simulink model "GridConnectedPVarray"  (R2024a)
settings: Solver=VariableStepAuto  StartTime=0.0  StopTime=1  RelTol=1e-3
libraries: spsSeriesRLCBranchLib x13, spsDiodeLib x7, spsIGBTDiodeLib x7, spsMeanLib x3, spsThreePhaseVIMeasurementLib x3, spsVoltageMeasurementLib x2, slpidlib x2, spsCurrentMeasurementLib x1, spsPVArrayLib x1, simulink x1, eeGeneralControl x1, spsThreePhaseSourceLib x1
settings Model: Creator=aditl  LastModifiedBy=aditl

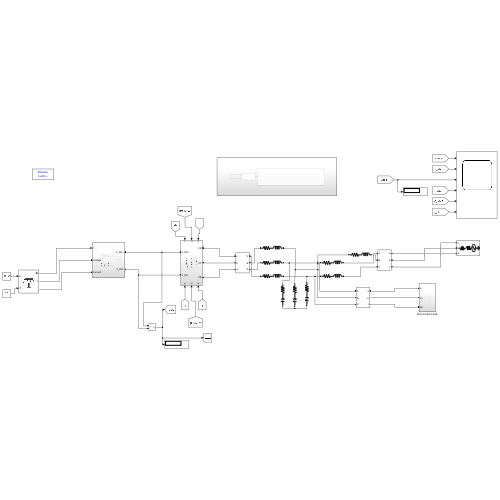
[thumbnail: Simulink's stored preview of the top-level diagram]
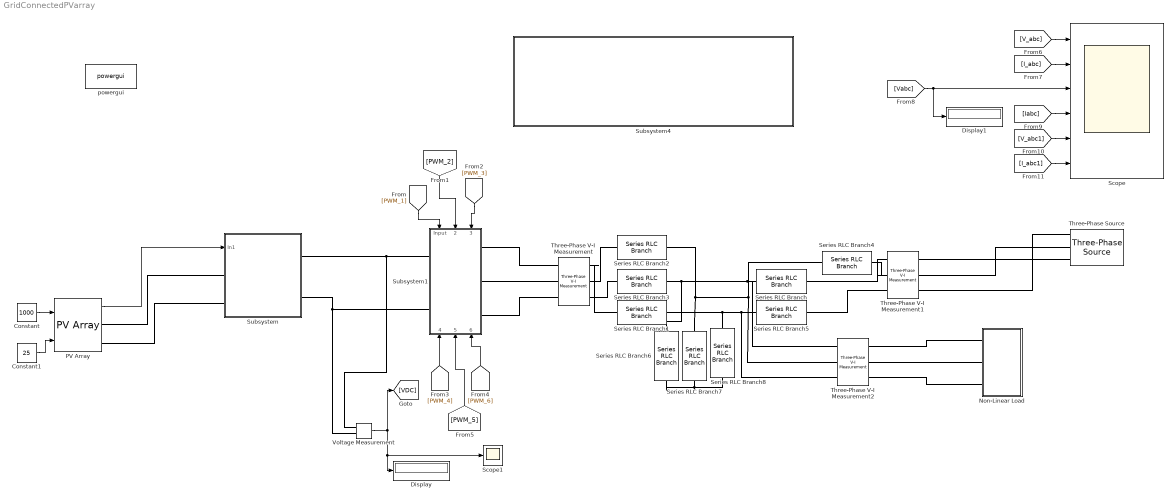
== system GridConnectedPVarray ==
  Constant : Constant  Value=1000
  Constant1 : Constant  Value=25
  Display : Display
  Display1 : Display
  Non-Linear Load : Subsystem
  PV Array : spsPVArrayLib/PV Array  Npar=40  Nser=10  PlotType=array @ 1000 W/m2 & specified temperatures  S_vec="[ 1000  500  100 ]"  Temp_C_vec="[ 45 25  ]"  ModuleName=User-defined  PlotWhenSelected=off  Pm=213.15  Ncell=60  Voc=36.3  Isc=7.84  Vm=29  Im=7.35  beta_Voc_pc=-0.36099  alpha_Isc_pc=0.102  beta_Voc=-0.13104  alpha_Isc=0.0079968  IL=7.8654  I0=2.9273e-10  nI=0.98119  Rsh=313.0553  Rs=0.39381  RobustModel=off  RobustCellTemperature=313.3991  BAL=on  Tc=1e-6  Tfilter=5e-5
  Scope : Scope  NumInputPorts=6
  Scope1 : Scope
  Series RLC Branch{,1..5} (6 alike) : spsSeriesRLCBranchLib/Series RLC Branch  LConnTagsString=__new0  RConnTagsString=__new0  BranchType=RL  Resistance=1e-3  Inductance=500e-6  SetiL0=off  InitialCurrent=0  Capacitance=1e-6  Setx0=off  InitialVoltage=0  Measurements=None
  Series RLC Branch6 : spsSeriesRLCBranchLib/Series RLC Branch  LConnTagsString=__new0  RConnTagsString=__new0  BranchType=RC  Resistance=1e-3  Inductance=1e-3  SetiL0=off  InitialCurrent=0  Capacitance=100e-6  Setx0=off  InitialVoltage=0  Measurements=None
  Series RLC Branch7 : spsSeriesRLCBranchLib/Series RLC Branch  LConnTagsString=__new0  RConnTagsString=__new0  BranchType=RC  Resistance=1e-3  Inductance=1e-3  SetiL0=off  InitialCurrent=0  Capacitance=100e-6  Setx0=off  InitialVoltage=0  Measurements=None
  Series RLC Branch8 : spsSeriesRLCBranchLib/Series RLC Branch  LConnTagsString=__new0  RConnTagsString=__new0  BranchType=RC  Resistance=1e-3  Inductance=1e-3  SetiL0=off  InitialCurrent=0  Capacitance=100e-6  Setx0=off  InitialVoltage=0  Measurements=None
  Subsystem : Subsystem
  Subsystem1 : Subsystem
      settings: PortSchema="{\"entries\":[{\"content\":{\"sides\":[{\"content\":{\"connectorIds\":[\"LConn1\",\"LConn2\"]},\"type\":\"ConnectorPlacement.EquallySpacedRectSide\",\"uuid\":\"a2a7ddac-ae87-4c1a-8b74-688f39786139\"},{\"content\":{\"connectorIds\":[\"RConn1\",\"RConn2\",\"RConn3\"],\"side\":\"RIGHT\"},\"type\":\"ConnectorPlacement.EquallySpacedRectSide\",\"uuid\":\"0ffaccab-b326-455c-8204-264bcaba31f0\"},{\"content\":{\"connectorIds\":[\"In1\",\"In2\",\"In3\"],\"side\":\"TOP\"},\"type\":\"ConnectorPlacement.EquallySpacedRectSide\",\"uuid\":\"7b315db4-04ed-4dc6-88af-8ad8e918cdd7\"},{\"content\":{\"connectorIds\":[\"In4\",\"In5\",\"In6\"],\"side\":\"BOTTOM\"},\"type\":\"ConnectorPlacement.EquallySpacedRectSide\",\"uuid\":\"b8aad6e0-d398-4abc-9931-0eadad765190\"}]},\"type\":\"ConnectorPlacement.EquallySpacedConnector\",\"uuid\":\"72918063-f98b-4253-8381-9410a0d32035\"}],\"packageUris\":[\"http://schema.mathworks.com/mf0/Connector/R2020b\"],\"version\":\"1.0\"}"
  Subsystem4 : Subsystem
  Three-Phase V-I Measurement : spsThreePhaseVIMeasurementLib/Three-Phase V-I Measurement  VoltageMeasurement=phase-to-ground  SetLabelV=on  LabelV=V_abc  Vpu=off  VpuLL=off  CurrentMeasurement=yes  SetLabelI=on  LabelI=I_abc  Ipu=off  Pbase=100e6  Vbase=500e3  OutputType=Complex  PhasorSimulation=off  PSBequivalent=0
  Three-Phase V-I Measurement1 : spsThreePhaseVIMeasurementLib/Three-Phase V-I Measurement  VoltageMeasurement=phase-to-ground  SetLabelV=on  LabelV=Vabc  Vpu=off  VpuLL=off  CurrentMeasurement=yes  SetLabelI=on  LabelI=Iabc  Ipu=off  Pbase=100e6  Vbase=500e3  OutputType=Complex  PhasorSimulation=off  PSBequivalent=0
  Three-Phase V-I Measurement2 : spsThreePhaseVIMeasurementLib/Three-Phase V-I Measurement  VoltageMeasurement=phase-to-ground  SetLabelV=on  LabelV=V_abc1  Vpu=off  VpuLL=off  CurrentMeasurement=yes  SetLabelI=on  LabelI=I_abc1  Ipu=off  Pbase=100e6  Vbase=500e3  OutputType=Complex  PhasorSimulation=off  PSBequivalent=0
  Three-Phase Source : spsThreePhaseSourceLib/Three-Phase Source  InternalConnection=Yg  VoltagePhases=off  Voltage=415  PhaseAngle=0  Voltage_phases=[25e3 25e3 25e3]/sqrt(3)  PhaseAngles_phases=[0 -120 +120]  Frequency=50  NonIdealSource=on  SpecifyImpedance=off  Resistance=1e-6  Inductance=1e6  ShortCircuitLevel=100e6  BaseVoltage=400  XRratio=7  BusType=swing  Pref=10e3  Qref=0  Prefabc=[10e3, 10e3, 10e3]  Qrefabc=[0, 0, 0]  Qmin=-inf  Qmax=inf
  Voltage Measurement : spsVoltageMeasurementLib/Voltage Measurement  PhasorSimulation=off  OutputType=Complex  PSBequivalent=0
  powergui : spspowerguiLib/powergui  Priority=1  SimulationMode=Discrete  SampleTime=1e-06  frequency=60  Iterations=50  frequencyindice=0  Pbase=100e6  ErrMax=1e-4  UnitsV=kV  UnitsW=MW  buscounter=0  FunctionMessages=off  echomessages=off  EnableUseOfTLC=off  CurrentSourceSwitches=off  DisableSnubberDevices=off  DisableRonSwitches=off  DisableVfSwitches=off  DisplayEquations=off  AutomaticDiscreteSolvers=off  SolverType=Tustin/Backward Euler (TBE)  Interpol=off  ExternalGateDelay=off  methode=off  Ts=100  x0status=blocks  SPID=on  SwTol=0  HookPort=off  NonlinearTolerance=0  nMaxIteration=15  ContinueOnMaxIteration=off  RestoreLinks=warning  ResistiveCurrentMeasurement=off  Frange=[0:2:500]  Ylog=off  Xlog=on  ShowGrid=off  save=off  variable=ZData  structure=0  ZoomFFT=off  StartTime=0.0  cycles=1  DisplayStyle=1  fundamental=60  FreqAxis=off  MaxFrequency=1000  frequencyindicesteady=1  RmsSteady=1  display=off
  wires:
  Constant/1 -> PV Array/1
  Constant1/1 -> PV Array/2
  PV Array/1 -> Subsystem/1(In1)
  [PWM_1] -> Subsystem1/1(Input)
  [PWM_2] -> Subsystem1/2(Input1)
  [PWM_3] -> Subsystem1/3(Input2)
  [PWM_4] -> Subsystem1/4(Input3)
  [PWM_6] -> Subsystem1/6(Input4)
  [PWM_5] -> Subsystem1/5(Input5)
  [V_abc] -> Scope/1
  [I_abc] -> Scope/2
  [Vabc] -> Display1/1, Scope/3
  [Iabc] -> Scope/4
  [V_abc1] -> Scope/5
  [I_abc1] -> Scope/6
  Voltage Measurement/1 -> Scope1/1, Display/1, [VDC]
  connections:
  PV Array/RConn1 -- Subsystem/LConn1
  PV Array/RConn2 -- Subsystem/LConn2
  Subsystem1/LConn1 -- Voltage Measurement/LConn1 -- Subsystem/RConn1
  Subsystem1/LConn2 -- Voltage Measurement/LConn2 -- Subsystem/RConn2
  Series RLC Branch5/LConn1 -- Three-Phase V-I Measurement2/LConn3 -- Series RLC Branch8/LConn1 -- Series RLC Branch1/RConn1
  Series RLC Branch4/LConn1 -- Series RLC Branch7/LConn1 -- Series RLC Branch2/RConn1 -- Three-Phase V-I Measurement2/LConn2
  Series RLC Branch/LConn1 -- Three-Phase V-I Measurement2/LConn1 -- Series RLC Branch6/LConn1 -- Series RLC Branch3/RConn1
  Three-Phase V-I Measurement/RConn1 -- Subsystem1/RConn3
  Three-Phase V-I Measurement/RConn2 -- Subsystem1/RConn2
  Three-Phase V-I Measurement/RConn3 -- Subsystem1/RConn1
  Three-Phase V-I Measurement1/LConn1 -- Series RLC Branch/RConn1
  Three-Phase V-I Measurement1/LConn2 -- Series RLC Branch4/RConn1
  Three-Phase V-I Measurement1/LConn3 -- Series RLC Branch5/RConn1
  Series RLC Branch6/RConn1 -- Series RLC Branch7/RConn1 -- Series RLC Branch8/RConn1
  Three-Phase V-I Measurement2/RConn1 -- Non-Linear Load/LConn1
  Three-Phase V-I Measurement2/RConn2 -- Non-Linear Load/LConn2
  Three-Phase V-I Measurement2/RConn3 -- Non-Linear Load/LConn3
  Three-Phase V-I Measurement1/RConn1 -- Three-Phase Source/RConn1
  Three-Phase V-I Measurement1/RConn2 -- Three-Phase Source/RConn2
  Three-Phase Source/RConn3 -- Three-Phase V-I Measurement1/RConn3
  Three-Phase V-I Measurement/LConn1 -- Series RLC Branch3/LConn1
  Three-Phase V-I Measurement/LConn2 -- Series RLC Branch2/LConn1
  Three-Phase V-I Measurement/LConn3 -- Series RLC Branch1/LConn1

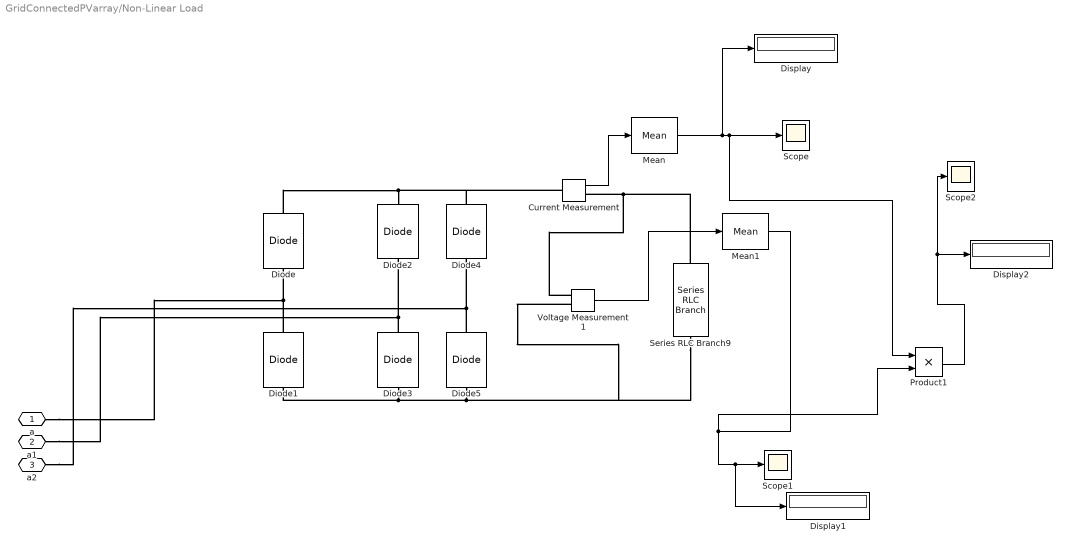
== system GridConnectedPVarray/Non-Linear Load ==
  Current Measurement : spsCurrentMeasurementLib/Current Measurement  PhasorSimulation=off  OutputType=Complex  PSBequivalent=0
  Diode{,1..5} (6 alike) : spsDiodeLib/Diode  Ron=0.001  Lon=0  Vf=0.8  IC=0  UseSnubber=0  Rs=500  Cs=250e-9  Measurements=off
  Display : Display
  Display1 : Display
  Display2 : Display
  Mean : spsMeanLib/Mean  Freq=60  Vinit=0  Ts=0
  Mean1 : spsMeanLib/Mean  Freq=60  Vinit=0  Ts=0
  Product1 : Product
  Scope : Scope
  Scope1 : Scope
  Scope2 : Scope
  Series RLC Branch9 : spsSeriesRLCBranchLib/Series RLC Branch  LConnTagsString=__new0  RConnTagsString=__new0  BranchType=RL  Resistance=31.23  Inductance=10e-3  SetiL0=off  InitialCurrent=0  Capacitance=1e-6  Setx0=off  InitialVoltage=0  Measurements=None
  Voltage Measurement1 : spsVoltageMeasurementLib/Voltage Measurement  PhasorSimulation=off  OutputType=Complex  PSBequivalent=0
  a : PMIOPort  Side=Left
  a1 : PMIOPort  Port=2  Side=Left
  a2 : PMIOPort  Port=3  Side=Left
  wires:
  Product1/1 -> Scope2/1, Display2/1
  Mean/1 -> Product1/1, Scope/1, Display/1
  Mean1/1 -> Display1/1, Scope1/1, Product1/2
  Voltage Measurement1/1 -> Mean1/1
  Current Measurement/1 -> Mean/1
  connections:
  Diode/RConn1 -- Current Measurement/LConn1 -- Diode4/RConn1 -- Diode2/RConn1
  Diode1/RConn1 -- Diode/LConn1 -- a/RConn1
  Diode3/LConn1 -- Voltage Measurement1/LConn2 -- Series RLC Branch9/RConn1 -- Diode5/LConn1 -- Diode1/LConn1
  Diode3/RConn1 -- Diode2/LConn1 -- a1/RConn1
  Diode5/RConn1 -- a2/RConn1 -- Diode4/LConn1
  Series RLC Branch9/LConn1 -- Voltage Measurement1/LConn1 -- Current Measurement/RConn1

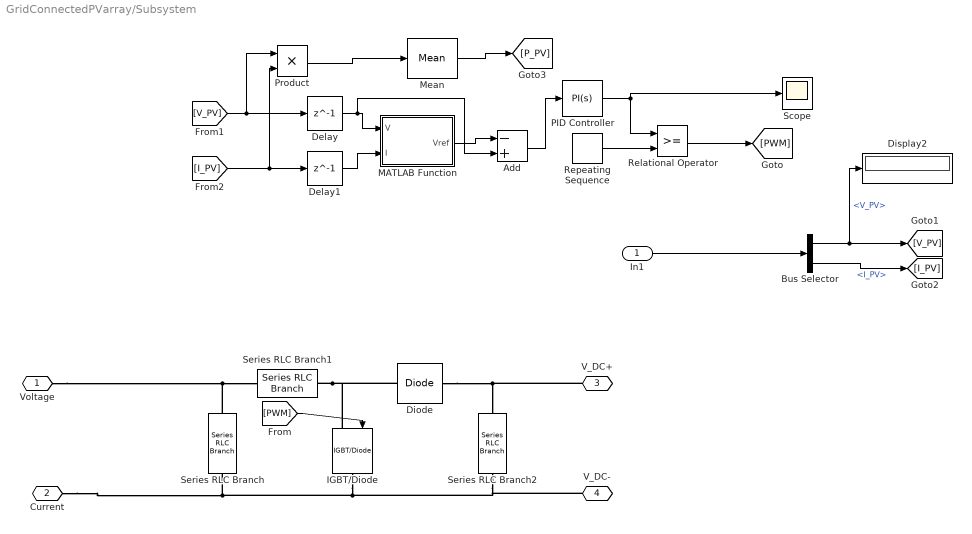
== system GridConnectedPVarray/Subsystem ==
  In1 : Inport
  Add : Sum  Inputs=-+
  Bus Selector : BusSelector  OutputSignals=V_PV,I_PV
  Delay : Delay  DelayLength=1  InitialCondition=0
  Delay1 : Delay  DelayLength=1  InitialCondition=0
  Diode : spsDiodeLib/Diode  Ron=0.001  Lon=2.2e-3  Vf=0.7  IC=0  UseSnubber=0  Rs=10e3  Cs=inf  Measurements=off
  Display2 : Display
  IGBT/Diode : spsIGBTDiodeLib/IGBT//Diode  Ron=.001  Rs=1e3  Cs=inf  Measurements=off
  MATLAB Function : MATLAB Function  TreatAsAtomicUnit=on
  Mean : spsMeanLib/Mean  Freq=60  Vinit=0  Ts=0
  PID Controller : slpidlib/PID Controller  Controller=PI  Form=Parallel  TimeDomain=Continuous-time  UseExternalTs=off  SampleTime=-1  IntegratorMethod=Forward Euler  FilterMethod=Forward Euler  ControllerParametersSource=internal  P=0.005  I=0.001  UseKiTs=off  D=0  UseExternalDerivativeSource=off  N=100  UseFilter=on  TunerSelectOption=Transfer Function Based (PID Tuner App)  InitialConditionSource=internal  InitialConditionForIntegrator=0  InitialConditionForFilter=0  DifferentiatorICPrevScaledInput=0  ExternalReset=none  TrackingMode=off  Kt=1  LimitOutput=on  SatLimitsSource=internal  UpperSaturationLimit=0.95  LowerSaturationLimit=0.00  LinearizeAsGain=on  AntiWindupMode=none  Kb=1  LimitIntegrator=off  UpperIntegratorSaturationLimit=inf  LowerIntegratorSaturationLimit=-inf  POutMin=[]  POutMax=[]  IOutMin=[]  IOutMax=[]  DOutMin=[]  DOutMax=[]  NOutMin=[]  NOutMax=[]  SumOutMin=[]  SumOutMax=[]  SaturationOutMin=[]  SaturationOutMax=[]  PParamMin=[]  PParamMax=[]  IParamMin=[]  IParamMax=[]  DParamMin=[]  DParamMax=[]  NParamMin=[]  NParamMax=[]  KbParamMin=[]  KbParamMax=[]  KtParamMin=[]  KtParamMax=[]  KbOutMin=[]  KbOutMax=[]  KtOutMin=[]  KtOutMax=[]  IntegratorOutMin=[]  IntegratorOutMax=[]  FilterOutMin=[]  FilterOutMax=[]  SumI1OutMin=[]  SumI1OutMax=[]  SumI2OutMin=[]  SumI2OutMax=[]  SumI3OutMin=[]  SumI3OutMax=[]  SumI4OutMin=[]  SumI4OutMax=[]  SumDOutMin=[]  SumDOutMax=[]  DifferentiatorOutMin=[]  DifferentiatorOutMax=[]  FilterDiffOutCoefMin=[]  FilterDiffOutCoefMax=[]  ReciprocalOutMin=[]  ReciprocalOutMax=[]  SumDenOutMin=[]  SumDenOutMax=[]  SumNumOutMin=[]  SumNumOutMax=[]  DivideOutMin=[]  DivideOutMax=[]  UdiffTsProdOutMin=[]  UdiffTsProdOutMax=[]  NTsProdOutMin=[]  NTsProdOutMax=[]  UintegralTsProdOutMin=[]  UintegralTsProdOutMax=[]  UngainTsProdOutMin=[]  UngainTsProdOutMax=[]  ClampingZeroOutDataTypeStr=Inherit: Inherit via back propagation  ClampingZeroOutMin=[]  ClampingZeroOutMax=[]  FilterDenConstantOutDataTypeStr=Inherit: Inherit via back propagation  FilterDenConstantOutMin=[]  FilterDenConstantOutMax=[]  PCopyOutDataTypeStr=Inherit: Inherit via back propagation  PCopyOutMin=[]  PCopyOutMax=[]  NCopyOutDataTypeStr=Inherit: Inherit via back propagation  NCopyOutMin=[]  NCopyOutMax=[]  IntegratorContinuousStateAttributes=''  IntegratorStateMustResolveToSignalObject=off  IntegratorRTWStateStorageClass=Auto  FilterContinuousStateAttributes=''  FilterStateMustResolveToSignalObject=off  FilterRTWStateStorageClass=Auto  ParallelPVariant=InternalParameters  IdealPVariant=Disabled  IVariant=InternalParameters  DVariant=Disabled  IntegratorVariant=Continuous  SatVariant=Enabled  AWVariant=Passthrough  PCopyVariant=Disabled  TRVariant=Disabled  FdbkBlocksVariant=Forward  IdealPFdbkVariant=Disabled  SatFdbkVariant=Disabled  DerivativeFilterVariant=Disabled  NVariant=Disabled  NCopyVariant=Disabled_SignalSpec  FilterICVariant=Disabled  IntegratorICVariant=InternalICs  ExternalResetVariant=Disabled  TRSumVariant=Passthrough  SumFdbkVariant=Disabled  SumVariant=Sum_PI  TsampFilterVariant=InternalTs  TsampNgainVariant=Passthrough  TsampIntegralVariant=Disabled_SignalSpec  ExternalSaturationOutDataTypeStr=Inherit: Same as second input  DerivativeSourceVariant=Disabled
  Product : Product
  Relational Operator : RelationalOperator  OutDataTypeStr=boolean  RndMeth=Simplest  InputSameDT=off
  Repeating Sequence : simulink/Sources/Repeating Sequence  rep_seq_t=[0 1/5000 ]  rep_seq_y=[0 1]
  Scope : Scope
  Series RLC Branch : spsSeriesRLCBranchLib/Series RLC Branch  LConnTagsString=__new0  RConnTagsString=__new0  BranchType=RC  Resistance=1e-6  Inductance=1e-3  SetiL0=off  InitialCurrent=0  Capacitance=1000e-6  Setx0=off  InitialVoltage=0  Measurements=None
  Series RLC Branch1 : spsSeriesRLCBranchLib/Series RLC Branch  LConnTagsString=__new0  RConnTagsString=__new0  BranchType=L  Resistance=1  Inductance=1.45e-3  SetiL0=off  InitialCurrent=0  Capacitance=1e-6  Setx0=off  InitialVoltage=0  Measurements=None
  Series RLC Branch2 : spsSeriesRLCBranchLib/Series RLC Branch  LConnTagsString=__new0  RConnTagsString=__new0  BranchType=C  Resistance=1  Inductance=1e-3  SetiL0=off  InitialCurrent=0  Capacitance=3227e-6  Setx0=off  InitialVoltage=0  Measurements=None
  Voltage : PMIOPort  Side=Left
  Current : PMIOPort  Port=2  Side=Left
  V_DC+ : PMIOPort  Port=3  Side=Right
  V_DC- : PMIOPort  Port=4  Side=Right
  wires:
  [V_PV] -> Product/1, Delay/1
  [I_PV] -> Product/2, Delay1/1
  Repeating Sequence/1 -> Relational Operator/2
  Mean/1 -> [P_PV]
  Add/1 -> PID Controller/1
  Delay/1 -> Add/2, MATLAB Function/1(V)
  Product/1 -> Mean/1
  Bus Selector/1 -> Display2/1, [V_PV]  "<V_PV>"
  MATLAB Function/1(Vref) -> Add/1
  PID Controller/1 -> Relational Operator/1, Scope/1
  Relational Operator/1 -> [PWM]
  Delay1/1 -> MATLAB Function/2(I)
  Bus Selector/2 -> [I_PV]  "<I_PV>"
  [PWM] -> IGBT/Diode/1
  In1/1 -> Bus Selector/1
  connections:
  Diode/RConn1 -- V_DC+/RConn1 -- Series RLC Branch2/LConn1
  Series RLC Branch1/LConn1 -- IGBT/Diode/LConn1 -- Diode/LConn1
  IGBT/Diode/RConn1 -- V_DC-/RConn1 -- Series RLC Branch2/RConn1 -- Current/RConn1 -- Series RLC Branch/RConn1
  Series RLC Branch/LConn1 -- Voltage/RConn1 -- Series RLC Branch1/RConn1

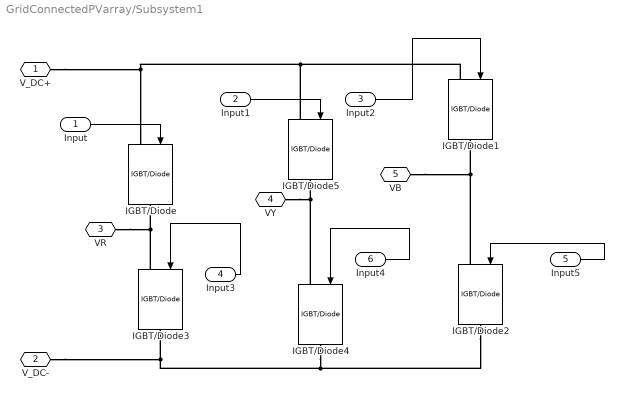
== system GridConnectedPVarray/Subsystem1 ==
  Input : Inport
  Input1 : Inport  Port=2
  Input2 : Inport  Port=3
  Input3 : Inport  Port=4
  Input5 : Inport  Port=5
  Input4 : Inport  Port=6
  IGBT/Diode{,1..5} (6 alike) : spsIGBTDiodeLib/IGBT//Diode  Ron=1e-3  Rs=1e5  Cs=inf  Measurements=off
  V_DC+ : PMIOPort  Side=Left
  V_DC- : PMIOPort  Port=2  Side=Left
  VR : PMIOPort  Port=3  Side=Right
  VY : PMIOPort  Port=4  Side=Right
  VB : PMIOPort  Port=5  Side=Right
  wires:
  Input2/1 -> IGBT/Diode1/1
  Input3/1 -> IGBT/Diode3/1
  Input1/1 -> IGBT/Diode5/1
  Input5/1 -> IGBT/Diode2/1
  Input4/1 -> IGBT/Diode4/1
  Input/1 -> IGBT/Diode/1
  connections:
  IGBT/Diode4/LConn1 -- VY/RConn1 -- IGBT/Diode5/RConn1
  IGBT/Diode1/LConn1 -- IGBT/Diode5/LConn1 -- V_DC+/RConn1 -- IGBT/Diode/LConn1
  IGBT/Diode2/LConn1 -- VB/RConn1 -- IGBT/Diode1/RConn1
  IGBT/Diode2/RConn1 -- IGBT/Diode4/RConn1 -- V_DC-/RConn1 -- IGBT/Diode3/RConn1
  IGBT/Diode3/LConn1 -- VR/RConn1 -- IGBT/Diode/RConn1

== system GridConnectedPVarray/Subsystem4 ==
  Subsystem2 : Subsystem
  Subsystem3 : Subsystem
  wires:
  [Vabc] -> Subsystem2/1(vs)
  Subsystem2/1(Is*) -> Subsystem3/1(In1)
  [Iabc] -> Subsystem2/2(Is)

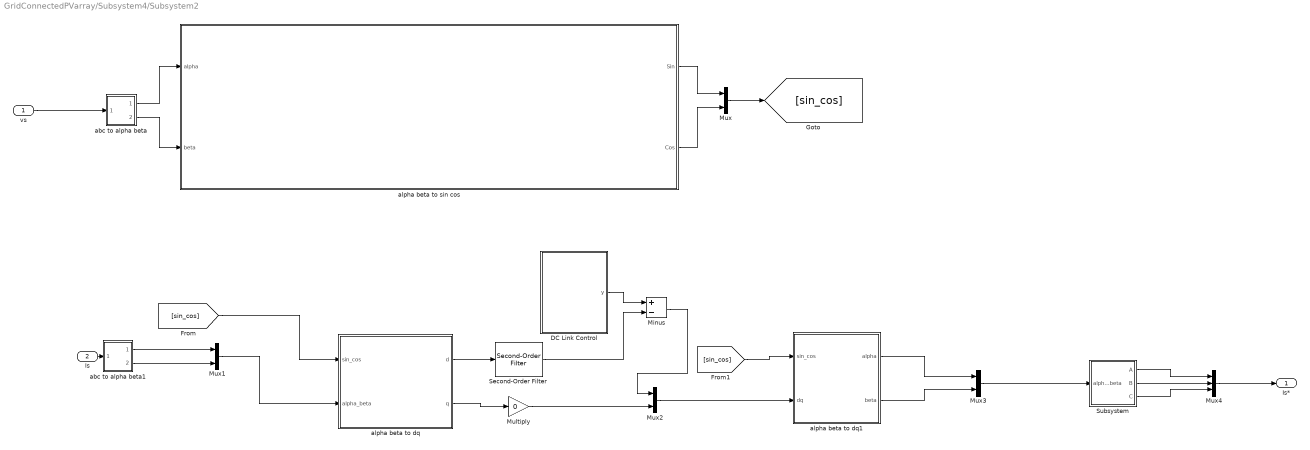
== system GridConnectedPVarray/Subsystem4/Subsystem2 ==
  vs : Inport
  Is : Inport  Port=2
  DC Link Control : Subsystem
  Minus : Sum  Inputs=+-
  Multiply : Gain  Gain=0
  Mux{,1..3} (4 alike) : Mux  Inputs=2
  Mux4 : Mux  Inputs=3
  Second-Order Filter : eeGeneralControl/Second-Order Filter  FilterType=Low-pass  fn=5  Zeta=0.707  Ts=1e-5  A0=0  Ph0=0  f0=0  b0=0
      settings: LibrarySourceBlock=ee_sl_lib/General Control/Second-Order Filter
  Subsystem : Subsystem
  abc to alpha beta : Subsystem
  abc to alpha beta1 : Subsystem
  alpha beta to dq : Subsystem
  alpha beta to dq1 : Subsystem
  alpha beta to sin cos : Subsystem
  Is* : Outport
  wires:
  abc to alpha beta/1(alpha) -> alpha beta to sin cos/1(alpha)
  abc to alpha beta/2(beta) -> alpha beta to sin cos/2(beta)
  alpha beta to sin cos/1(Sin) -> Mux/1
  alpha beta to sin cos/2(Cos) -> Mux/2
  Mux/1 -> [sin_cos]
  abc to alpha beta1/1(alpha) -> Mux1/1
  abc to alpha beta1/2(beta) -> Mux1/2
  [sin_cos] -> alpha beta to dq/1(sin_cos)
  Mux1/1 -> alpha beta to dq/2(alpha_beta)
  alpha beta to dq/1(d) -> Second-Order Filter/1
  alpha beta to dq/2(q) -> Multiply/1
  DC Link Control/1(y) -> Minus/1
  Second-Order Filter/1 -> Minus/2
  Minus/1 -> Mux2/1
  Multiply/1 -> Mux2/2
  Mux2/1 -> alpha beta to dq1/2(dq)
  [sin_cos] -> alpha beta to dq1/1(sin_cos)
  alpha beta to dq1/1(alpha) -> Mux3/1
  alpha beta to dq1/2(beta) -> Mux3/2
  Mux3/1 -> Subsystem/1(alpha_beta)
  Subsystem/1(A) -> Mux4/1
  Subsystem/2(B) -> Mux4/2
  Subsystem/3(C) -> Mux4/3
  vs/1 -> abc to alpha beta/1(In1)
  Is/1 -> abc to alpha beta1/1(In1)
  Mux4/1 -> Is*/1

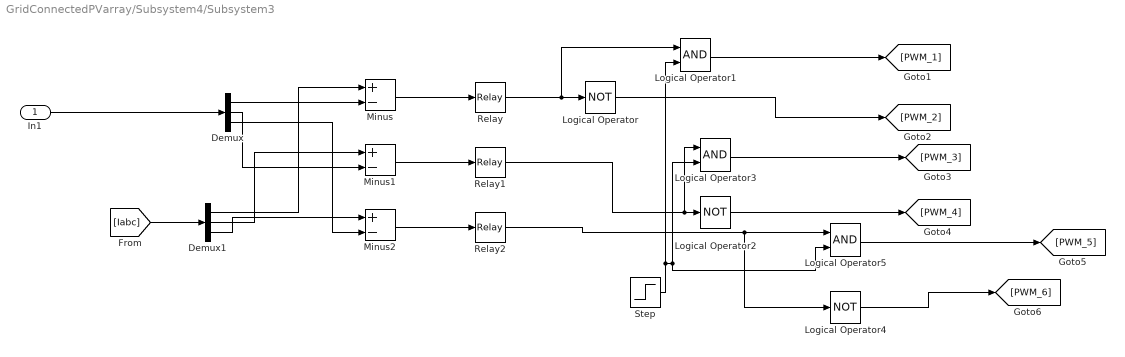
== system GridConnectedPVarray/Subsystem4/Subsystem3 ==
  In1 : Inport
  Demux : Demux  Outputs=3
  Demux1 : Demux  Outputs=3
  Logical Operator : Logic  Operator=NOT  AllPortsSameDT=off  OutDataTypeStr=boolean
  Logical Operator1 : Logic  AllPortsSameDT=off  OutDataTypeStr=boolean
  Logical Operator2 : Logic  Operator=NOT  AllPortsSameDT=off  OutDataTypeStr=boolean
  Logical Operator3 : Logic  AllPortsSameDT=off  OutDataTypeStr=boolean
  Logical Operator4 : Logic  Operator=NOT  AllPortsSameDT=off  OutDataTypeStr=boolean
  Logical Operator5 : Logic  AllPortsSameDT=off  OutDataTypeStr=boolean
  Minus : Sum  Inputs=+-
  Minus1 : Sum  Inputs=+-
  Minus2 : Sum  Inputs=+-
  Relay : Relay  OnSwitchValue=0.5  OffSwitchValue=-0.5
  Relay1 : Relay  OnSwitchValue=0.5  OffSwitchValue=-0.5
  Relay2 : Relay  OnSwitchValue=0.5  OffSwitchValue=-0.5
  Step : Step  SampleTime=0
  wires:
  Demux/3 -> Minus2/2
  Minus1/1 -> Relay1/1
  Step/1 -> Logical Operator5/2, Logical Operator3/2, Logical Operator1/2
  Logical Operator/1 -> [PWM_2]
  Relay2/1 -> Logical Operator4/1, Logical Operator5/1
  Demux/2 -> Minus1/2
  Logical Operator2/1 -> [PWM_4]
  Logical Operator3/1 -> [PWM_3]
  Demux1/2 -> Minus1/1
  Relay1/1 -> Logical Operator2/1, Logical Operator3/1
  Logical Operator5/1 -> [PWM_5]
  [Iabc] -> Demux1/1
  Logical Operator4/1 -> [PWM_6]
  Demux1/1 -> Minus/1
  In1/1 -> Demux/1
  Relay/1 -> Logical Operator1/1, Logical Operator/1
  Logical Operator1/1 -> [PWM_1]
  Minus/1 -> Relay/1
  Demux/1 -> Minus/2
  Minus2/1 -> Relay2/1
  Demux1/3 -> Minus2/1

== system GridConnectedPVarray/Subsystem4/Subsystem2/DC Link Control ==
  Constant : Constant  Value=686
  Minus : Sum  Inputs=+-
  PID Controller : slpidlib/PID Controller  Controller=PI  Form=Parallel  TimeDomain=Continuous-time  UseExternalTs=off  SampleTime=-1  IntegratorMethod=Forward Euler  FilterMethod=Forward Euler  ControllerParametersSource=internal  P=0.5  I=0.5  UseKiTs=off  D=0  UseExternalDerivativeSource=off  N=100  UseFilter=on  TunerSelectOption=Transfer Function Based (PID Tuner App)  InitialConditionSource=internal  InitialConditionForIntegrator=0  InitialConditionForFilter=0  DifferentiatorICPrevScaledInput=0  ExternalReset=none  TrackingMode=off  Kt=1  LimitOutput=off  SatLimitsSource=internal  UpperSaturationLimit=inf  LowerSaturationLimit=-inf  LinearizeAsGain=on  AntiWindupMode=none  Kb=1  LimitIntegrator=off  UpperIntegratorSaturationLimit=inf  LowerIntegratorSaturationLimit=-inf  POutMin=[]  POutMax=[]  IOutMin=[]  IOutMax=[]  DOutMin=[]  DOutMax=[]  NOutMin=[]  NOutMax=[]  SumOutMin=[]  SumOutMax=[]  SaturationOutMin=[]  SaturationOutMax=[]  PParamMin=[]  PParamMax=[]  IParamMin=[]  IParamMax=[]  DParamMin=[]  DParamMax=[]  NParamMin=[]  NParamMax=[]  KbParamMin=[]  KbParamMax=[]  KtParamMin=[]  KtParamMax=[]  KbOutMin=[]  KbOutMax=[]  KtOutMin=[]  KtOutMax=[]  IntegratorOutMin=[]  IntegratorOutMax=[]  FilterOutMin=[]  FilterOutMax=[]  SumI1OutMin=[]  SumI1OutMax=[]  SumI2OutMin=[]  SumI2OutMax=[]  SumI3OutMin=[]  SumI3OutMax=[]  SumI4OutMin=[]  SumI4OutMax=[]  SumDOutMin=[]  SumDOutMax=[]  DifferentiatorOutMin=[]  DifferentiatorOutMax=[]  FilterDiffOutCoefMin=[]  FilterDiffOutCoefMax=[]  ReciprocalOutMin=[]  ReciprocalOutMax=[]  SumDenOutMin=[]  SumDenOutMax=[]  SumNumOutMin=[]  SumNumOutMax=[]  DivideOutMin=[]  DivideOutMax=[]  UdiffTsProdOutMin=[]  UdiffTsProdOutMax=[]  NTsProdOutMin=[]  NTsProdOutMax=[]  UintegralTsProdOutMin=[]  UintegralTsProdOutMax=[]  UngainTsProdOutMin=[]  UngainTsProdOutMax=[]  ClampingZeroOutDataTypeStr=Inherit: Inherit via back propagation  ClampingZeroOutMin=[]  ClampingZeroOutMax=[]  FilterDenConstantOutDataTypeStr=Inherit: Inherit via back propagation  FilterDenConstantOutMin=[]  FilterDenConstantOutMax=[]  PCopyOutDataTypeStr=Inherit: Inherit via back propagation  PCopyOutMin=[]  PCopyOutMax=[]  NCopyOutDataTypeStr=Inherit: Inherit via back propagation  NCopyOutMin=[]  NCopyOutMax=[]  IntegratorContinuousStateAttributes=''  IntegratorStateMustResolveToSignalObject=off  IntegratorRTWStateStorageClass=Auto  FilterContinuousStateAttributes=''  FilterStateMustResolveToSignalObject=off  FilterRTWStateStorageClass=Auto  ParallelPVariant=InternalParameters  IdealPVariant=Disabled  IVariant=InternalParameters  DVariant=Disabled  IntegratorVariant=Continuous  SatVariant=Disabled  AWVariant=Passthrough  PCopyVariant=Disabled  TRVariant=Disabled  FdbkBlocksVariant=Forward  IdealPFdbkVariant=Disabled  SatFdbkVariant=Disabled  DerivativeFilterVariant=Disabled  NVariant=Disabled  NCopyVariant=Disabled_SignalSpec  FilterICVariant=Disabled  IntegratorICVariant=InternalICs  ExternalResetVariant=Disabled  TRSumVariant=Passthrough  SumFdbkVariant=Disabled  SumVariant=Sum_PI  TsampFilterVariant=InternalTs  TsampNgainVariant=Passthrough  TsampIntegralVariant=Disabled_SignalSpec  ExternalSaturationOutDataTypeStr=Inherit: Same as second input  DerivativeSourceVariant=Disabled
  y : Outport
  wires:
  [Vdc] -> Minus/2
  Constant/1 -> Minus/1
  Minus/1 -> PID Controller/1
  PID Controller/1 -> y/1

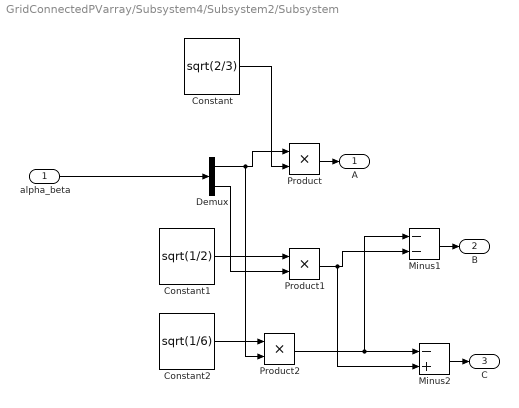
== system GridConnectedPVarray/Subsystem4/Subsystem2/Subsystem ==
  alpha_beta : Inport
  Constant : Constant  Value=sqrt(2/3)
  Constant1 : Constant  Value=sqrt(1/2)
  Constant2 : Constant  Value=sqrt(1/6)
  Demux : Demux  Outputs=2
  Minus1 : Sum  Inputs=--
  Minus2 : Sum  Inputs=-+
  Product : Product
  Product1 : Product
  Product2 : Product
  A : Outport
  B : Outport  Port=2
  C : Outport  Port=3
  wires:
  Constant/1 -> Product/2
  Demux/2 -> Product1/2
  Product2/1 -> Minus1/1, Minus2/1
  Demux/1 -> Product2/2, Product/1
  Product1/1 -> Minus2/2, Minus1/2
  Product/1 -> A/1
  Constant2/1 -> Product2/1
  Minus2/1 -> C/1
  Constant1/1 -> Product1/1
  Minus1/1 -> B/1
  alpha_beta/1 -> Demux/1

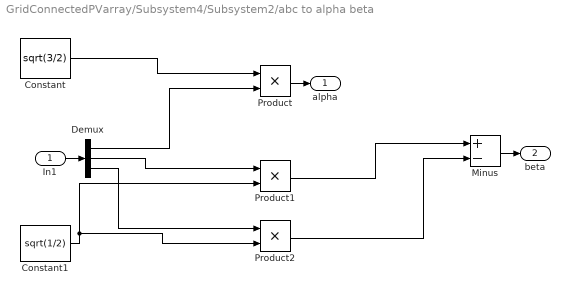
== system GridConnectedPVarray/Subsystem4/Subsystem2/abc to alpha beta ==
  In1 : Inport
  Constant : Constant  Value=sqrt(3/2)
  Constant1 : Constant  Value=sqrt(1/2)
  Demux : Demux  Outputs=3
  Minus : Sum  Inputs=+-
  Product : Product
  Product1 : Product
  Product2 : Product
  alpha : Outport
  beta : Outport  Port=2
  wires:
  Demux/3 -> Product2/1
  Constant1/1 -> Product1/2, Product2/2
  Constant/1 -> Product/1
  In1/1 -> Demux/1
  Product2/1 -> Minus/2
  Product1/1 -> Minus/1
  Demux/2 -> Product1/1
  Demux/1 -> Product/2
  Minus/1 -> beta/1
  Product/1 -> alpha/1

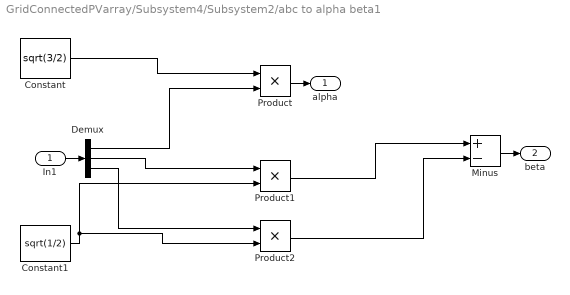
== system GridConnectedPVarray/Subsystem4/Subsystem2/abc to alpha beta1 ==
  In1 : Inport
  Constant : Constant  Value=sqrt(3/2)
  Constant1 : Constant  Value=sqrt(1/2)
  Demux : Demux  Outputs=3
  Minus : Sum  Inputs=+-
  Product : Product
  Product1 : Product
  Product2 : Product
  alpha : Outport
  beta : Outport  Port=2
  wires:
  Demux/3 -> Product2/1
  Constant1/1 -> Product1/2, Product2/2
  Constant/1 -> Product/1
  In1/1 -> Demux/1
  Product2/1 -> Minus/2
  Product1/1 -> Minus/1
  Demux/2 -> Product1/1
  Demux/1 -> Product/2
  Minus/1 -> beta/1
  Product/1 -> alpha/1

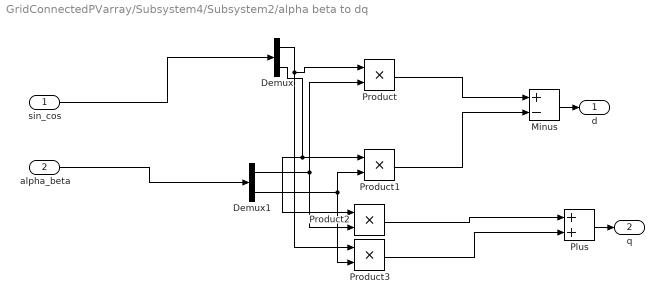
== system GridConnectedPVarray/Subsystem4/Subsystem2/alpha beta to dq ==
  sin_cos : Inport
  alpha_beta : Inport  Port=2
  Demux : Demux  Outputs=2
  Demux1 : Demux  Outputs=2
  Minus : Sum  Inputs=+-
  Plus : Sum
  Product{,1..3} (4 alike) : Product
  d : Outport
  q : Outport  Port=2
  wires:
  Demux/1 -> Product3/1, Product/1
  Product2/1 -> Plus/1
  Product3/1 -> Plus/2
  Demux/2 -> Product2/1, Product1/1
  Demux1/2 -> Product1/2, Product3/2
  Product1/1 -> Minus/2
  Demux1/1 -> Product/2, Product2/2
  sin_cos/1 -> Demux/1
  Product/1 -> Minus/1
  alpha_beta/1 -> Demux1/1
  Plus/1 -> q/1
  Minus/1 -> d/1

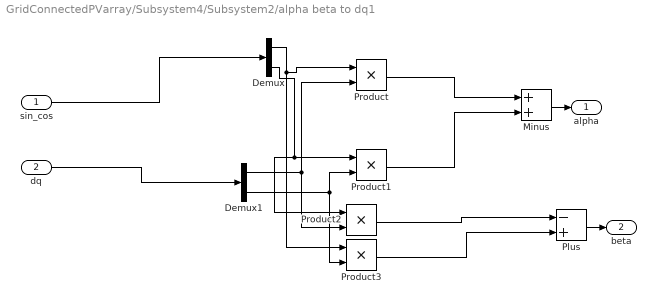
== system GridConnectedPVarray/Subsystem4/Subsystem2/alpha beta to dq1 ==
  sin_cos : Inport
  dq : Inport  Port=2
  Demux : Demux  Outputs=2
  Demux1 : Demux  Outputs=2
  Minus : Sum
  Plus : Sum  Inputs=-+
  Product{,1..3} (4 alike) : Product
  alpha : Outport
  beta : Outport  Port=2
  wires:
  Demux/1 -> Product3/1, Product/1
  Product2/1 -> Plus/1
  Product3/1 -> Plus/2
  Demux/2 -> Product2/1, Product1/1
  Demux1/2 -> Product1/2, Product3/2
  Product1/1 -> Minus/2
  Demux1/1 -> Product/2, Product2/2
  sin_cos/1 -> Demux/1
  Product/1 -> Minus/1
  dq/1 -> Demux1/1
  Plus/1 -> beta/1
  Minus/1 -> alpha/1

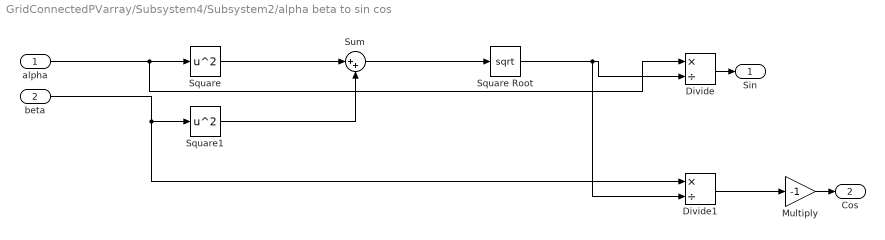
== system GridConnectedPVarray/Subsystem4/Subsystem2/alpha beta to sin cos ==
  alpha : Inport
  beta : Inport  Port=2
  Divide : Product  Inputs=*/
  Divide1 : Product  Inputs=*/
  Multiply : Gain  Gain=-1
  Square : Math  Operator=square
  Square Root : Sqrt
  Square1 : Math  Operator=square
  Sum : Sum  Inputs=|++
  Sin : Outport
  Cos : Outport  Port=2
  wires:
  Square/1 -> Sum/1
  Divide/1 -> Sin/1
  Square Root/1 -> Divide1/2, Divide/2
  Square1/1 -> Sum/2
  alpha/1 -> Divide/1, Square/1
  Divide1/1 -> Multiply/1
  Sum/1 -> Square Root/1
  beta/1 -> Divide1/1, Square1/1
  Multiply/1 -> Cos/1

== matlab function GridConnectedPVarray/Subsystem/MATLAB Function ==
  data: V input; Vref output; I input
function Vref = RefGen(V,I)
 
Vrefmax=363;
Vrefmin=0;
Vrefinit=300;
deltaVref=1;
persistent Vold Pold Vrefold;
 
dataType = 'double';
 
if isempty(Vold)
    Vold=0;
    Pold=0;
    Vrefold=Vrefinit;
end
 
P=V*I;
dV=V-Vold;
dP=P-Pold;
 
if dP~=0
    if dP<0
        if dV<0
            Vref=Vrefold+deltaVref;
        else
            Vref=Vrefold-deltaVref;
        end
    else
        if dV<0
            Vref=Vrefold-deltaVref;
        else
            Vref=Vrefold+deltaVref;
        end
    end
else
    Vref=Vrefold;
end
 
if Vref>=Vrefmax | Vref<= Vrefmin
    Vref=Vrefold;
end
 
Vrefold=Vref;
Vold=V;
Pold=P;
